simulink model "sampleModel1756"  (R2023a)
settings: Solver=VariableStepAuto  StartTime=0.0  StopTime=10.0  RelTol=1e-3
libraries: hdlsllib x5
settings Model: Creator=user1  LastModifiedBy=user1

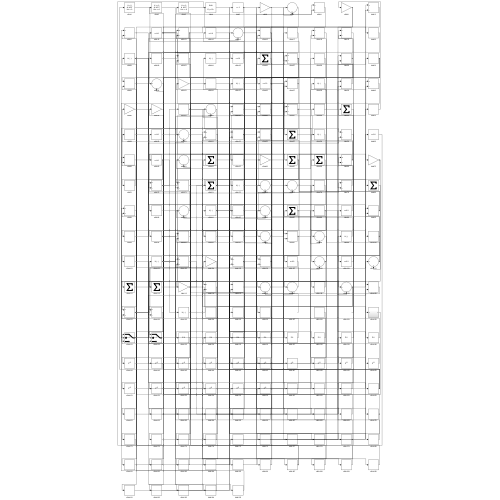
[thumbnail: Simulink's stored preview of the top-level diagram]
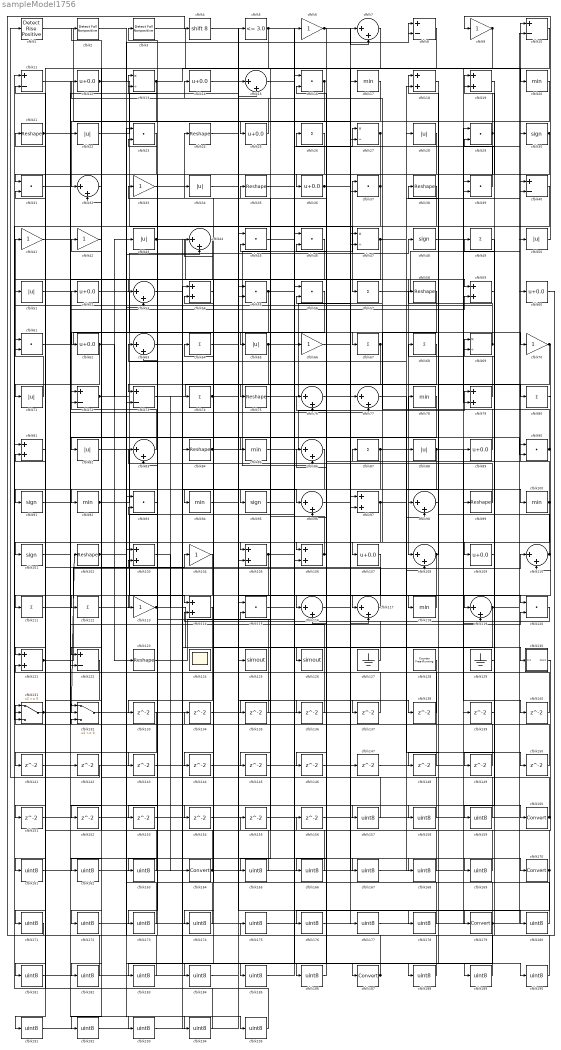
== system sampleModel1756 ==
  cfblk1 : hdlsllib/Logic and Bit Operations/Detect Rise Positive  vinit=0  OutDataTypeStr=boolean
  cfblk{8,10..11,40,72..73,122} (7 alike) : Sum  Inputs=+-
  cfblk{17,20,78,85,92,94,100,118} (8 alike) : MinMax
  cfblk{30,48,91,95,101} (5 alike) : Signum
  cfblk{21,24,35,38,58,75,84,99,102,123} (10 alike) : Reshape
  cfblk{18..19,54,59,79,81,97,103,105..106,114,121} (12 alike) : Sum
  cfblk{6,9,33,41..42,66,70,104,113} (9 alike) : Gain
  cfblk{12,14,25,36,52,60,62,89,107,109} (10 alike) : Bias  Bias=0.0  SaturateOnIntegerOverflow=off
  cfblk{7,15,32,44,53,63,76..77,83,86,96,98,108,110,116..117,119} (17 alike) : Sum  Inputs=|++
  cfblk{26,49,57,64,67..68,74,80,87,111..112} (11 alike) : Sum  Inputs=+
  cfblk{16,23,29,31,37,39,45..46,55..56,61,90,93,115,120} (15 alike) : DotProduct  OutDataTypeStr=Inherit: Inherit via internal rule
  cfblk124 : Scope
      settings: Floating=on
  cfblk125 : ToWorkspace  VariableName=simout  SaveFormat=Timeseries  SampleTime=-1
  cfblk126 : ToWorkspace  VariableName=simout  SaveFormat=Timeseries  SampleTime=-1
  cfblk127 : Ground
  cfblk128 : hdlsllib/Sources/Counter Free-Running  NumBits=16  tsamp=-1
  cfblk129 : Ground
  cfblk{13,27,47,69} (4 alike) : Product  Inputs=*/  RndMeth=Zero  SaturateOnIntegerOverflow=on
  cfblk130 : Subsystem
      settings: LibrarySourceBlock=|
      | hdlsllib/Ports &
      | Subsystems/Subsystem
  cfblk131 : Switch  SaturateOnIntegerOverflow=off  InputSameDT=off
  cfblk132 : Switch  SaturateOnIntegerOverflow=off  InputSameDT=off
  cfblk{133..156} (24 alike) : Delay  SampleTime=1
  cfblk{157..159,161..163,165..169,171..178,180..186,188..195} (34 alike) : DataTypeConversion  OutDataTypeStr=uint8  SaturateOnIntegerOverflow=off  RndMeth=Floor
  cfblk{160,164,170,179,187} (5 alike) : DataTypeConversion  SaturateOnIntegerOverflow=off  RndMeth=Floor
  cfblk2 : hdlsllib/Logic and Bit Operations/Detect Fall Nonpositive  vinit=0  OutDataTypeStr=boolean
  cfblk{22,28,34,43,50..51,65,71,82,88} (10 alike) : Abs  SaturateOnIntegerOverflow=off
  cfblk3 : hdlsllib/Logic and Bit Operations/Detect Fall Nonpositive  vinit=0  OutDataTypeStr=boolean
  cfblk4 : ArithShift  BitShiftNumber=8
  cfblk5 : hdlsllib/Logic and Bit Operations/Compare To Constant  relop=<=  const=3.0  OutDataTypeStr=boolean
  wires:
  cfblk29/1 -> cfblk19/1, cfblk53/1
  cfblk19/1 -> cfblk36/1
  cfblk83/1 -> cfblk52/1
  cfblk72/1 -> cfblk43/1, cfblk28/1
  cfblk121/1 -> cfblk110/1, cfblk59/2, cfblk169/1
  cfblk70/1 -> cfblk117/1, cfblk98/1
  cfblk6/1 -> cfblk116/1, cfblk7/2
  cfblk84/1 -> cfblk37/1, cfblk86/2
  cfblk100/1 -> cfblk10/1, cfblk33/1, cfblk171/1, cfblk176/1
  cfblk108/1 -> cfblk118/1, cfblk18/1
  cfblk28/1 -> cfblk106/1
  cfblk85/1 -> cfblk79/1
  cfblk110/1 -> cfblk109/1, cfblk87/1
  cfblk109/1 -> cfblk49/1
  cfblk64/1 -> cfblk179/1
  cfblk17/1 -> cfblk32/1
  cfblk71/1 -> cfblk41/1
  cfblk123/1 -> cfblk56/1
  cfblk69/1 -> cfblk51/1, cfblk58/1
  cfblk82/1 -> cfblk114/1
  cfblk4/1 -> cfblk170/1
  cfblk50/1 -> cfblk9/1
  cfblk92/1 -> cfblk48/1, cfblk185/1
  cfblk41/1 -> cfblk59/1
  cfblk87/1 -> cfblk150/1, cfblk151/1
  cfblk113/1 -> cfblk126/1, cfblk74/1
  cfblk12/1 -> cfblk57/1, cfblk8/2, cfblk195/1
  cfblk132/1 -> cfblk106/2
  cfblk106/1 -> cfblk35/1, cfblk146/1
  cfblk51/1 -> cfblk13/1
  cfblk63/1 -> cfblk187/1
  cfblk80/1 -> cfblk110/2
  cfblk112/1 -> cfblk6/1
  cfblk33/1 -> cfblk24/1
  cfblk61/1 -> cfblk67/1
  cfblk103/1 -> cfblk164/1
  cfblk47/1 -> cfblk91/1, cfblk40/2
  cfblk16/1 -> cfblk105/1, cfblk85/1
  cfblk75/1 -> cfblk17/1
  cfblk118/1 -> cfblk111/1
  cfblk128/1 -> cfblk131/1
  cfblk52/1 -> cfblk70/1
  cfblk86/1 -> cfblk92/1
  cfblk30/1 -> cfblk62/1, cfblk96/2, cfblk73/1
  cfblk117/1 -> cfblk21/1
  cfblk131/1 -> cfblk102/1, cfblk120/2
  cfblk91/1 -> cfblk22/1
  cfblk99/1 -> cfblk83/1
  cfblk88/1 -> cfblk122/1, cfblk140/1
  cfblk73/1 -> cfblk80/1
  cfblk26/1 -> cfblk95/1
  cfblk120/1 -> cfblk114/2
  cfblk48/1 -> cfblk30/1
  cfblk57/1 -> cfblk40/1
  cfblk107/1 -> cfblk131/2
  cfblk116/1 -> cfblk37/2
  cfblk7/1 -> cfblk116/2
  cfblk127/1 -> cfblk76/1
  cfblk10/1 -> cfblk79/2
  cfblk111/1 -> cfblk104/1
  cfblk58/1 -> cfblk107/1
  cfblk74/1 -> cfblk54/2, cfblk119/1, cfblk138/1
  cfblk8/1 -> cfblk25/1
  cfblk97/1 -> cfblk98/2, cfblk192/1
  cfblk9/1 -> cfblk82/1, cfblk165/1
  cfblk35/1 -> cfblk27/1
  cfblk43/1 -> cfblk108/1, cfblk96/1
  cfblk37/1 -> cfblk113/1, cfblk31/1
  cfblk40/1 -> cfblk83/2
  cfblk20/1 -> cfblk72/2
  cfblk22/1 -> cfblk5/1
  cfblk129/1 -> cfblk69/1
  cfblk54/1 -> cfblk94/1
  cfblk14/1 -> cfblk125/1
  cfblk93/1 -> cfblk3/1
  cfblk39/1 -> cfblk26/1
  cfblk67/1 -> cfblk135/1, cfblk174/1
  cfblk65/1 -> cfblk75/1, cfblk119/2
  cfblk1/1 -> cfblk97/1
  cfblk96/1 -> cfblk78/1
  cfblk77/1 -> cfblk100/1
  cfblk53/1 -> cfblk130/1(In1)
  cfblk119/1 -> cfblk50/1, cfblk144/1, cfblk166/1
  cfblk5/1 -> cfblk120/1, cfblk161/1
  cfblk44/1 -> cfblk61/2
  cfblk56/1 -> cfblk132/1
  cfblk38/1 -> cfblk131/3
  cfblk66/1 -> cfblk160/1
  cfblk25/1 -> cfblk14/1
  cfblk32/1 -> cfblk112/1
  cfblk21/1 -> cfblk71/1, cfblk76/2, cfblk90/2
  cfblk36/1 -> cfblk69/2, cfblk168/1
  cfblk27/1 -> cfblk101/1, cfblk65/1, cfblk145/1
  cfblk102/1 -> cfblk44/2, cfblk53/2, cfblk154/1
  cfblk76/1 -> cfblk7/1
  cfblk55/1 -> cfblk8/1, cfblk153/1
  cfblk89/1 -> cfblk12/1
  cfblk62/1 -> cfblk132/2, cfblk123/1, cfblk121/1
  cfblk2/1 -> cfblk27/2
  cfblk13/1 -> cfblk20/1, cfblk73/2, cfblk182/1
  cfblk105/1 -> cfblk77/2, cfblk122/2
  cfblk90/1 -> cfblk56/2, cfblk68/1
  cfblk79/1 -> cfblk38/1
  cfblk3/1 -> cfblk47/2
  cfblk104/1 -> cfblk133/1
  cfblk134/1 -> cfblk47/1
  cfblk135/1 -> cfblk13/2
  cfblk34/1 -> cfblk136/1
  cfblk136/1 -> cfblk16/1
  cfblk94/1 -> cfblk137/1
  cfblk137/1 -> cfblk54/1
  cfblk138/1 -> cfblk93/2
  cfblk139/1 -> cfblk19/2
  cfblk140/1 -> cfblk61/1
  cfblk122/1 -> cfblk141/1
  cfblk141/1 -> cfblk77/1
  cfblk31/1 -> cfblk142/1
  cfblk142/1 -> cfblk1/1
  cfblk114/1 -> cfblk143/1
  cfblk144/1 -> cfblk108/2
  cfblk145/1 -> cfblk117/2
  cfblk146/1 -> cfblk97/2
  cfblk147/1 -> cfblk29/1
  cfblk98/1 -> cfblk148/1
  cfblk148/1 -> cfblk44/1
  cfblk49/1 -> cfblk149/1
  cfblk149/1 -> cfblk72/1
  cfblk150/1 -> cfblk86/1
  cfblk151/1 -> cfblk18/2
  cfblk78/1 -> cfblk152/1
  cfblk154/1 -> cfblk105/2
  cfblk130/1(Out1) -> cfblk155/1
  cfblk155/1 -> cfblk10/2
  cfblk45/1 -> cfblk157/1
  cfblk157/1 -> cfblk34/1
  cfblk101/1 -> cfblk158/1
  cfblk158/1 -> cfblk45/1
  cfblk59/1 -> cfblk159/1
  cfblk159/1 -> cfblk45/2
  cfblk160/1 -> cfblk134/1, cfblk132/3, cfblk2/1, cfblk16/2
  cfblk161/1 -> cfblk66/1
  cfblk42/1 -> cfblk162/1
  cfblk162/1 -> cfblk147/1
  cfblk68/1 -> cfblk163/1
  cfblk163/1 -> cfblk42/1
  cfblk164/1 -> cfblk139/1, cfblk31/2, cfblk88/1
  cfblk165/1 -> cfblk103/1
  cfblk166/1 -> cfblk103/2
  cfblk115/1 -> cfblk167/1
  cfblk167/1 -> cfblk99/1
  cfblk168/1 -> cfblk115/1
  cfblk169/1 -> cfblk115/2
  cfblk170/1 -> cfblk32/2, cfblk186/1
  cfblk171/1 -> cfblk4/1
  cfblk23/1 -> cfblk172/1
  cfblk172/1 -> cfblk89/1
  cfblk143/1 -> cfblk173/1
  cfblk173/1 -> cfblk23/1
  cfblk174/1 -> cfblk23/2
  cfblk60/1 -> cfblk175/1
  cfblk175/1 -> cfblk90/1
  cfblk176/1 -> cfblk60/1
  cfblk156/1 -> cfblk177/1
  cfblk177/1 -> cfblk39/2
  cfblk95/1 -> cfblk178/1
  cfblk178/1 -> cfblk156/1
  cfblk179/1 -> cfblk39/1, cfblk183/1
  cfblk24/1 -> cfblk180/1
  cfblk180/1 -> cfblk64/1
  cfblk81/1 -> cfblk181/1
  cfblk181/1 -> cfblk55/1
  cfblk182/1 -> cfblk81/1
  cfblk183/1 -> cfblk81/2
  cfblk46/1 -> cfblk184/1
  cfblk184/1 -> cfblk55/2
  cfblk185/1 -> cfblk46/1
  cfblk186/1 -> cfblk46/2
  cfblk187/1 -> cfblk121/2, cfblk93/1
  cfblk18/1 -> cfblk188/1
  cfblk188/1 -> cfblk63/1
  cfblk153/1 -> cfblk189/1
  cfblk189/1 -> cfblk63/2
  cfblk15/1 -> cfblk190/1
  cfblk190/1 -> cfblk29/2
  cfblk133/1 -> cfblk191/1
  cfblk191/1 -> cfblk15/1
  cfblk192/1 -> cfblk15/2
  cfblk11/1 -> cfblk193/1
  cfblk193/1 -> cfblk84/1
  cfblk152/1 -> cfblk194/1
  cfblk194/1 -> cfblk11/1
  cfblk195/1 -> cfblk11/2

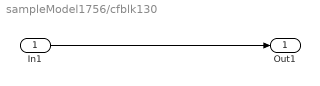
== system sampleModel1756/cfblk130 ==
  In1 : Inport
  Out1 : Outport
  wires:
  In1/1 -> Out1/1
